simulink model "test_steady_state_manager7_7"  (R2020b)
settings: Solver=VariableStepAuto  StartTime=0.0  StopTime=10.0  RelTol=1e-3
values from neighbouring files (symbols this model uses):
  g = 9.81    [Esercizio7_7_Matlab.m]    (also in Setup_SIM.m)
  gamma0 = convang(0.000,'deg','rad')    [Esercizio7_7_Matlab.m]    (also in Setup_SIM.m)
  myAC = DSVAircraft(aircraftDataFileName)    [Esercizio7_7_Matlab.m]    (also in Setup_SIM.m)
  q0 = convangvel(0.000,'deg/s','rad/s')    [Esercizio7_7_Matlab.m]    (also in Setup_SIM.m)
  V0 = 320.0    (= 320)    [Setup_SIM.m]
  xEG_0 = 0    [Esercizio7_7_Matlab.m]    (also in Setup_SIM.m)
  zEG_0 = -4000    [Esercizio7_7_Matlab.m]    (also in Setup_SIM.m)
libraries: aerolibatmos2 x1
settings Model: Creator=Andrea  LastModifiedBy=isido

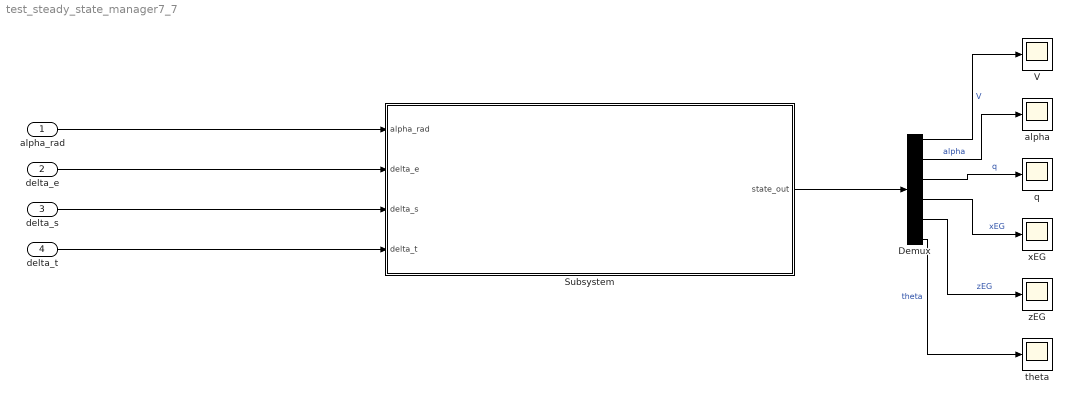
== system test_steady_state_manager7_7 ==
  alpha_rad : Inport
  delta_e : Inport  Port=2
  delta_s : Inport  Port=3
  delta_t : Inport  Port=4
  Demux : Demux  Outputs=6
  Subsystem : Subsystem
  V : Scope
  alpha : Scope
  q : Scope
  theta : Scope
  xEG : Scope
  zEG : Scope
  wires:
  Demux/1 -> V/1  "V"
  delta_t/1 -> Subsystem/4(delta_t)
  Subsystem/1(state_out) -> Demux/1
  alpha_rad/1 -> Subsystem/1(alpha_rad)
  Demux/3 -> q/1  "q"
  Demux/5 -> zEG/1  "zEG"
  Demux/6 -> theta/1  "theta"
  Demux/4 -> xEG/1  "xEG"
  Demux/2 -> alpha/1  "alpha"
  delta_s/1 -> Subsystem/3(delta_s)
  delta_e/1 -> Subsystem/2(delta_e)

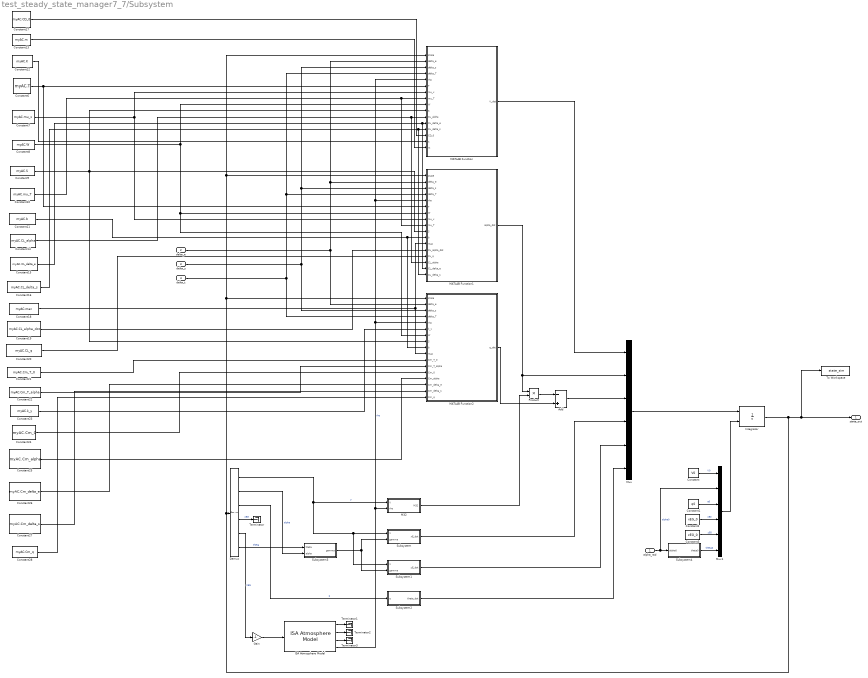
== system test_steady_state_manager7_7/Subsystem ==
  alpha_rad : Inport
  delta_e : Inport  Port=2
  delta_s : Inport  Port=3
  delta_t : Inport  Port=4
  Add : Sum  Inputs=-+
  Constant : Constant  Value=V0
  Constant1 : Constant  Value=q0
  Constant10 : Constant  Value=myAC.mu_T
  Constant11 : Constant  Value=myAC.b
  Constant12 : Constant  Value=myAC.K
  Constant13 : Constant  Value=myAC.m
  Constant14 : Constant  Value=myAC.CL_alpha
  Constant15 : Constant  Value=myAC.CL_delta_e
  Constant16 : Constant  Value=myAC.CL_delta_s
  Constant17 : Constant  Value=myAC.CD_0
  Constant18 : Constant  Value=myAC.mac
  Constant19 : Constant  Value=myAC.CL_alpha_dot
  Constant2 : Constant  Value=xEG_0
  Constant20 : Constant  Value=myAC.CL_q
  Constant21 : Constant  Value=myAC.Cm_T_0
  Constant22 : Constant  Value=myAC.Cm_T_alpha
  Constant23 : Constant  Value=myAC.k_y
  Constant24 : Constant  Value=myAC.Cm_0
  Constant25 : Constant  Value=myAC.Cm_alpha
  Constant26 : Constant  Value=myAC.Cm_delta_e
  Constant27 : Constant  Value=myAC.Cm_delta_s
  Constant28 : Constant  Value=myAC.Cm_q
  Constant3 : Constant  Value=zEG_0
  Constant6 : Constant  Value=myAC.T
  Constant7 : Constant  Value=myAC.mu_x
  Constant8 : Constant  Value=myAC.W
  Constant9 : Constant  Value=myAC.S
  Demux : Demux  Outputs=6
  Gain : Gain  Gain=-1
  ISA Atmosphere Model : aerolibatmos2/ISA Atmosphere Model  custom=off  g=9.80665  gamma=1.4  R=287.0531  L=0.0065  h_trop=11000  h_strat=20000  rho0=1.225  P0=101325  T0=288.15  h0=0
  Integrator : Integrator  InitialConditionSource=external
  M32 : Subsystem
  MATLAB Function : MATLAB Function  TreatAsAtomicUnit=on
  MATLAB Function1 : MATLAB Function  TreatAsAtomicUnit=on
  MATLAB Function2 : MATLAB Function  TreatAsAtomicUnit=on
  Mux : Mux  Inputs=6
  Mux1 : Mux  Inputs=6
  Product : Product
  Subsystem : Subsystem
  Subsystem1 : Subsystem
  Subsystem2 : Subsystem
  Subsystem3 : Subsystem
  Subsystem4 : Subsystem
  Terminator{,1..3} (4 alike) : Terminator
  To Workspace : ToWorkspace  VariableName=state_sim  SaveFormat=Timeseries  SampleTime=-1
  state_out : Outport
  wires:
  MATLAB Function/1(V_dot) -> Mux/1
  MATLAB Function1/1(alpha_dot) -> Product/1, Mux/2
  Add/1 -> Mux/3
  MATLAB Function2/1(q_dot) -> Add/2
  M32/1(M32) -> Product/2
  Product/1 -> Add/1
  Subsystem/1(xE_dot) -> Mux/4
  Subsystem1/1(zE_dot) -> Mux/5
  Subsystem2/1(theta_dot) -> Mux/6
  Subsystem3/1(gamma) -> Subsystem1/2(gamma), Subsystem/2(gamma)
  Mux/1 -> Integrator/1
  Mux1/1 -> Integrator/2
  Constant/1 -> Mux1/1  "V0"
  alpha_rad/1 -> Mux1/2, Subsystem4/1(alpha0)  "alpha0"
  Constant1/1 -> Mux1/3  "q0"
  Constant2/1 -> Mux1/4  "xE0"
  Constant3/1 -> Mux1/5  "zE0"
  Subsystem4/1(theta0) -> Mux1/6  "theta0"
  delta_e/1 -> MATLAB Function2/2(delta_e), MATLAB Function/2(delta_e), MATLAB Function1/2(delta_e)
  delta_s/1 -> MATLAB Function2/3(delta_s), MATLAB Function/3(delta_s), MATLAB Function1/3(delta_s)
  delta_t/1 -> MATLAB Function2/4(delta_T), MATLAB Function/4(delta_T), MATLAB Function1/4(delta_T)
  Integrator/1 -> MATLAB Function/1(state), MATLAB Function1/1(state), MATLAB Function2/1(state), Demux/1, To Workspace/1, state_out/1
  Demux/1 -> Subsystem1/1(V), Subsystem/1(V), M32/1(V)  "V"
  Demux/3 -> Subsystem2/1(q)  "q"
  Demux/6 -> Subsystem3/1(theta)  "theta"
  Demux/2 -> Subsystem3/2(alpha)  "alpha"
  Demux/4 -> Terminator/1  "xEG"
  Demux/5 -> Gain/1  "zEG"
  Gain/1 -> ISA Atmosphere Model/1
  ISA Atmosphere Model/1 -> Terminator1/1
  ISA Atmosphere Model/2 -> Terminator2/1
  ISA Atmosphere Model/3 -> Terminator3/1
  ISA Atmosphere Model/4 -> MATLAB Function/5(rho), MATLAB Function1/5(rho), MATLAB Function2/5(rho), M32/2(rho)  "rho"
  Constant6/1 -> MATLAB Function1/6(T), MATLAB Function/6(T)
  Constant7/1 -> MATLAB Function1/8(mu_x), MATLAB Function/7(mu_x)
  Constant8/1 -> MATLAB Function2/7(W), MATLAB Function1/7(W), MATLAB Function/9(W)
  Constant9/1 -> MATLAB Function2/8(S), MATLAB Function1/10(S), MATLAB Function/10(S)
  Constant10/1 -> MATLAB Function/8(mu_T), MATLAB Function1/9(mu_T)
  Constant11/1 -> MATLAB Function1/11(b), MATLAB Function2/9(b)
  Constant12/1 -> MATLAB Function/15(K)
  Constant13/1 -> MATLAB Function/16(m)
  Constant14/1 -> MATLAB Function/11(CL_alpha), MATLAB Function1/15(CL_alpha)
  Constant15/1 -> MATLAB Function1/16(CL_delta_e), MATLAB Function/12(CL_delta_e)
  Constant16/1 -> MATLAB Function/13(CL_delta_s), MATLAB Function1/17(CL_delta_s)
  Constant17/1 -> MATLAB Function/14(CD_0)
  Constant18/1 -> MATLAB Function2/10(mac), MATLAB Function1/12(mac)
  Constant19/1 -> MATLAB Function1/13(CL_alpha_dot)
  Constant20/1 -> MATLAB Function1/14(CL_q)
  Constant21/1 -> MATLAB Function2/11(Cm_T_0)
  Constant22/1 -> MATLAB Function2/12(Cm_T_alpha)
  Constant23/1 -> MATLAB Function2/6(k_y)
  Constant24/1 -> MATLAB Function2/13(Cm_0)
  Constant25/1 -> MATLAB Function2/14(Cm_alpha)
  Constant26/1 -> MATLAB Function2/15(Cm_delta_e)
  Constant27/1 -> MATLAB Function2/16(Cm_delta_s)
  Constant28/1 -> MATLAB Function2/17(Cm_q)

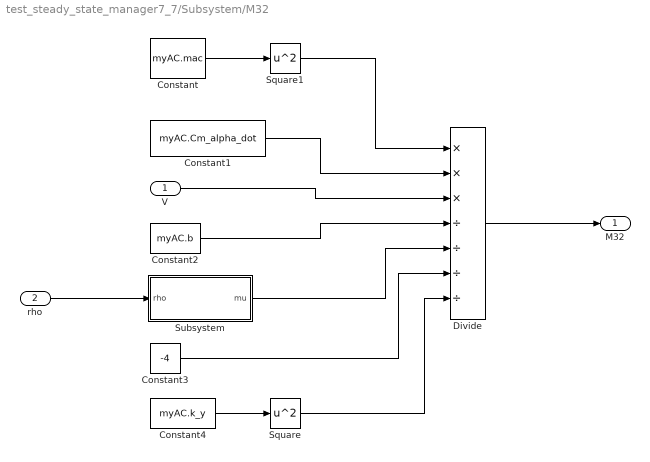
== system test_steady_state_manager7_7/Subsystem/M32 ==
  V : Inport
  rho : Inport  Port=2
  Constant : Constant  Value=myAC.mac
  Constant1 : Constant  Value=myAC.Cm_alpha_dot
  Constant2 : Constant  Value=myAC.b
  Constant3 : Constant  Value=-4
  Constant4 : Constant  Value=myAC.k_y
  Divide : Product  Inputs=***////
  Square : Math  Operator=square  SaturateOnIntegerOverflow=on
  Square1 : Math  Operator=square  SaturateOnIntegerOverflow=on
  Subsystem : Subsystem
  M32 : Outport
  wires:
  Constant/1 -> Square1/1
  Constant4/1 -> Square/1
  Square1/1 -> Divide/1
  Constant1/1 -> Divide/2
  V/1 -> Divide/3
  Constant2/1 -> Divide/4
  Subsystem/1(mu) -> Divide/5
  Constant3/1 -> Divide/6
  Square/1 -> Divide/7
  Divide/1 -> M32/1
  rho/1 -> Subsystem/1(rho)

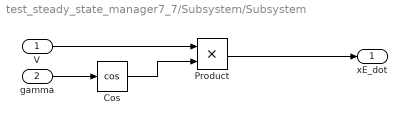
== system test_steady_state_manager7_7/Subsystem/Subsystem ==
  V : Inport
  gamma : Inport  Port=2
  Cos : Trigonometry  Operator=cos
  Product : Product
  xE_dot : Outport
  wires:
  gamma/1 -> Cos/1
  Cos/1 -> Product/2
  V/1 -> Product/1
  Product/1 -> xE_dot/1

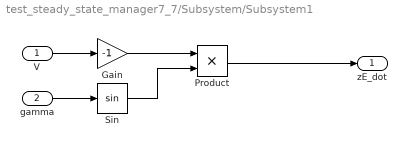
== system test_steady_state_manager7_7/Subsystem/Subsystem1 ==
  V : Inport
  gamma : Inport  Port=2
  Gain : Gain  Gain=-1
  Product : Product
  Sin : Trigonometry
  zE_dot : Outport
  wires:
  gamma/1 -> Sin/1
  Sin/1 -> Product/2
  V/1 -> Gain/1
  Product/1 -> zE_dot/1
  Gain/1 -> Product/1

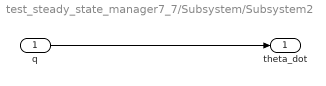
== system test_steady_state_manager7_7/Subsystem/Subsystem2 ==
  q : Inport
  theta_dot : Outport
  wires:
  q/1 -> theta_dot/1

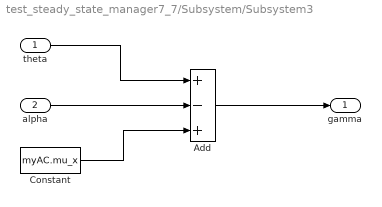
== system test_steady_state_manager7_7/Subsystem/Subsystem3 ==
  theta : Inport
  alpha : Inport  Port=2
  Add : Sum  Inputs=+-+
  Constant : Constant  Value=myAC.mu_x
  gamma : Outport
  wires:
  theta/1 -> Add/1
  alpha/1 -> Add/2
  Constant/1 -> Add/3
  Add/1 -> gamma/1

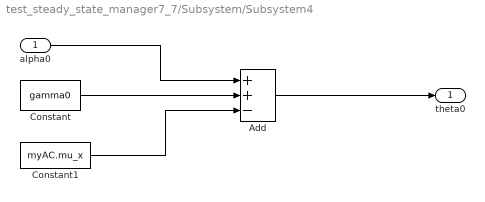
== system test_steady_state_manager7_7/Subsystem/Subsystem4 ==
  alpha0 : Inport
  Add : Sum  Inputs=++-
  Constant : Constant  Value=gamma0
  Constant1 : Constant  Value=myAC.mu_x
  theta0 : Outport
  wires:
  Constant/1 -> Add/2
  alpha0/1 -> Add/1
  Constant1/1 -> Add/3
  Add/1 -> theta0/1

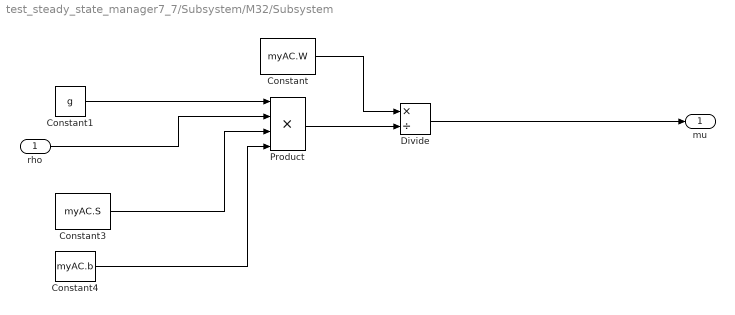
== system test_steady_state_manager7_7/Subsystem/M32/Subsystem ==
  rho : Inport
  Constant : Constant  Value=myAC.W
  Constant1 : Constant  Value=g
  Constant3 : Constant  Value=myAC.S
  Constant4 : Constant  Value=myAC.b
  Divide : Product  Inputs=*/
  Product : Product  Inputs=4
  mu : Outport
  wires:
  Divide/1 -> mu/1
  rho/1 -> Product/2
  Constant/1 -> Divide/1
  Product/1 -> Divide/2
  Constant1/1 -> Product/1
  Constant4/1 -> Product/4
  Constant3/1 -> Product/3

== matlab function test_steady_state_manager7_7/Subsystem/MATLAB Function1 ==
  data: state input; alpha_dot output; delta_e input; delta_s input; delta_T input; rho input; T input; W input; mu_x input; mu_T input; S input; b input; mac input; CL_alpha_dot input; CL_q input; CL_alpha input; CL_delta_e input; CL_delta_s input
function alpha_dot = fcn(state, delta_e,delta_s,delta_T,rho,T,W,mu_x,mu_T,S,b,mac,CL_alpha_dot,CL_q,CL_alpha,CL_delta_e,CL_delta_s)

g=9.81;

V = state(1);
alpha = state(2);
q = state(3);
xEG = state(4);
zEG = state(5);
theta = state(6);

T_over_W = T/W;
alphaB_plus_muT = alpha - mu_x + mu_T;
mu_rel = (W/g)/(rho*S*b); 
gamma_t = theta - alpha + mu_x;
macOverb_over_FourMuRel_dot_CLAlphadot = (mac/b)*CL_alpha_dot/(4*mu_rel);
macOverb_over_FourMuRel_dot_CLq = (mac/b)*CL_q/(4*mu_rel);
g_over_V = g/V;
rhoVsquare_over_TwoWeightSurface = rho*V^2/(2*(W/S));
CL_coeff = CL_alpha*alpha + CL_delta_e*delta_e+...
           CL_delta_s*delta_s;
alpha_dot = 1/(1 + macOverb_over_FourMuRel_dot_CLAlphadot)*...
            (q*(1 - macOverb_over_FourMuRel_dot_CLq)-...
               delta_T*(T_over_W)*(g_over_V)*sin(alphaB_plus_muT)+...
               (g_over_V)*cos(gamma_t)-...
               (rhoVsquare_over_TwoWeightSurface*g_over_V)*CL_coeff);

== matlab function test_steady_state_manager7_7/Subsystem/MATLAB Function ==
  data: state input; V_dot output; delta_e input; delta_s input; delta_T input; rho input; T input; mu_x input; mu_T input; W input; S input; CL_alpha input; CL_delta_e input; CL_delta_s input; CD_0 input; K input; m input
function V_dot = fcn(state, delta_e,delta_s,delta_T,rho,T,mu_x,mu_T,W,S,CL_alpha,CL_delta_e,CL_delta_s,CD_0,K,m)

g=9.81;

V = state(1);
alpha = state(2);
q = state(3);
xEG = state(4);
zEG = state(5);
theta = state(6);

T_over_W = T/W;
alphaB_plus_muT = alpha - mu_x + mu_T;
gamma_t = theta - alpha + mu_x;
rhoVsquare_over_TwoWeightSurface = rho*V^2/(2*(W/S));
CL_coeff = CL_alpha*alpha + CL_delta_e*delta_e+...
           CL_delta_s*delta_s;
V_dot = g*((delta_T*T_over_W)*cos(alphaB_plus_muT)-...
           sin(gamma_t) - (rhoVsquare_over_TwoWeightSurface)*...
                          (CD_0 + K*(CL_coeff)^m));

== matlab function test_steady_state_manager7_7/Subsystem/MATLAB Function2 ==
  data: state input; q_dot output; delta_e input; delta_s input; delta_T input; rho input; k_y input; W input; S input; b input; mac input; Cm_T_0 input; Cm_T_alpha input; Cm_0 input; Cm_alpha input; Cm_delta_e input; Cm_delta_s input; Cm_q input
function q_dot = fcn(state,delta_e,delta_s,delta_T,rho,k_y,W,S,b,mac,Cm_T_0,Cm_T_alpha,Cm_0,Cm_alpha,Cm_delta_e,Cm_delta_s,Cm_q)

g=9.81;

V = state(1);
alpha = state(2);
q = state(3);
xEG = state(4);
zEG = state(5);
theta = state(6);

V_over_radiusgirationSquared = (V/(k_y))^2;  
mu_rel = (W/g)/(rho*S*b); 
macOverb_over_TwoMuRel = (mac/b)/(2*mu_rel);
CM_T = (Cm_T_0 + Cm_T_alpha*alpha)*delta_T;
CM_coeff = Cm_0 + Cm_alpha*alpha + Cm_delta_e*delta_e+...
           Cm_delta_s*delta_s+...
           (mac/(2*V))*(Cm_q*q);        
q_dot = (V_over_radiusgirationSquared)*(macOverb_over_TwoMuRel)*...
        (CM_T + CM_coeff);
